simulink model "robot_rk"  (R2014b)
settings: Solver=ode45  StartTime=0.0  StopTime=10  FixedStep=1e-4  RelTol=1e-3
values from neighbouring files (symbols this model uses):
  robot_floor_friction_coeff = 0.6    [robot_init.m]
  robot_floor_position_gain = -1e5    (= -100000)    [robot_init.m]
  robot_floor_speed_gain = -1e3    (= -1000)    [robot_init.m]
  robot_gravity = [0 0 -9.80665]    [robot_init.m]
undefined symbols (not defined in the file or in its folder): CM730_acc_center, CM730_acc_gain, CM730_default, CM730_gyro_center, CM730_gyro_gain, CM730_sample_time, FSR_max, FSR_no_load, FSR_sample_time, FSR_scale, MX28_default, MX28_inertia, MX28_Te, X, Y, Z
libraries: sm_lib x158, fl_lib x128, nesl_utility x77
(part 6 of 6)

== system robot_rk/Right Leg/Floor model/Floor Model Front Right ==
  6-DOF Joint1 : sm_lib/Joints/6-DOF Joint  SenseConstraintForce=off  SenseConstraintForceX=off  SenseConstraintForceY=off  SenseConstraintForceZ=off  SenseConstraintTorque=off  SenseConstraintTorqueX=off  SenseConstraintTorqueY=off  SenseConstraintTorqueZ=off  SenseTotalForce=off  SenseTotalForceX=off  SenseTotalForceY=off  SenseTotalForceZ=off  SenseTotalTorque=off  SenseTotalTorqueX=off  SenseTotalTorqueY=off  SenseTotalTorqueZ=off  CompositeWrenchDir=FollowerOnBase  CompositeWrenchFrame=BaseFrame  PxEquilibriumPosition=0  PxEquilibriumPositionUnits=m  PxSpringStiffness=0  PxSpringStiffnessUnits=N/m  PxDampingCoefficient=0  PxDampingCoefficientUnits=N/(m/s)  PxTorqueActuationMode=InputTorque  PxMotionActuationMode=ComputedMotion  PxSensePosition=off  PxSenseVelocity=on  PxSenseAcceleration=off  PxSenseTorqueForce=off  PxPositionTargetValue=0  PxPositionTargetValueUnits=m  PxPositionTargetSpecify=off  PxPositionTargetPriority=High  PxVelocityTargetValue=0  PxVelocityTargetValueUnits=m/s  PxVelocityTargetSpecify=off  PxVelocityTargetPriority=High  PyEquilibriumPosition=0  PyEquilibriumPositionUnits=m  PySpringStiffness=0  PySpringStiffnessUnits=N/m  PyDampingCoefficient=0  PyDampingCoefficientUnits=N/(m/s)  PyTorqueActuationMode=InputTorque  PyMotionActuationMode=ComputedMotion  PySensePosition=off  PySenseVelocity=on  PySenseAcceleration=off  PySenseTorqueForce=off  PyPositionTargetValue=0  PyPositionTargetValueUnits=m  PyPositionTargetSpecify=off  PyPositionTargetPriority=High  PyVelocityTargetValue=0  PyVelocityTargetValueUnits=m/s  PyVelocityTargetSpecify=off  PyVelocityTargetPriority=High  PzEquilibriumPosition=0  PzEquilibriumPositionUnits=m  PzSpringStiffness=0  PzSpringStiffnessUnits=N/m  PzDampingCoefficient=0  PzDampingCoefficientUnits=N/(m/s)  PzTorqueActuationMode=InputTorque  PzMotionActuationMode=ComputedMotion  PzSensePosition=on  PzSenseVelocity=on  PzSenseAcceleration=off  PzSenseTorqueForce=off  PzPositionTargetValue=0  PzPositionTargetValueUnits=m  PzPositionTargetSpecify=off  PzPositionTargetPriority=High  PzVelocityTargetValue=0  PzVelocityTargetValueUnits=m/s  PzVelocityTargetSpecify=off  PzVelocityTargetPriority=High  SphDefPosRotationMethod=None  SphDefPosRotationAngleUnits=deg  SphDefPosRotationStandardAxis=+Z  SphDefPosRotationAngle=0.0  SphDefPosRotationArbitraryAxis=[0 0 1]  SphDefPosFollAlignAxisA=+X  SphDefPosBaseAlignAxisA=+Y  SphDefPosFollAlignAxisB=+Y  SphDefPosBaseAlignAxisB=+Z  SphDefPosRotationMatrix=[1 0 0; 0 1 0; 0 0 1]  SphEqPosRotationMethod=None  SphEqPosRotationAngleUnits=deg  SphEqPosRotationStandardAxis=+Z  SphEqPosRotationAngle=0.0  SphEqPosRotationArbitraryAxis=[0 0 1]  SphEqPosFollAlignAxisA=+X  SphEqPosBaseAlignAxisA=+Y  SphEqPosFollAlignAxisB=+Y  SphEqPosBaseAlignAxisB=+Z  SphEqPosRotationMatrix=[1 0 0; 0 1 0; 0 0 1]  SphSpringStiffness=0  SphSpringStiffnessUnits=N*m/deg  SphDampingCoefficient=0  SphDampingCoefficientUnits=N*m/(deg/s)  SphActuateTorqueX=off  SphActuateTorqueY=off  SphActuateTorqueZ=off  SphActuateTorque=off  SphTorqueActuationMode=NoTorque  SphMotionActuationMode=ComputedMotion  SphActuationFrame=BaseFrame  SphSensePosition=off  SphSenseVelocityX=off  SphSenseVelocityY=off  SphSenseVelocityZ=off  SphSenseVelocity=off  SphSenseAccelerationX=off  SphSenseAccelerationY=off  SphSenseAccelerationZ=off  SphSenseAcceleration=off  SphSenseTorqueX=off  SphSenseTorqueY=off  SphSenseTorqueZ=off  SphSenseTorqueForce=off  SphSensingFrame=BaseFrame  SphPositionTargetRotationMethod=None  SphPositionTargetRotationAngleUnits=deg  SphPositionTargetRotationStandardAxis=+Z  SphPositionTargetRotationAngle=0.0  SphPositionTargetRotationArbitraryAxis=[0 0 1]  SphPositionTargetFollAlignAxisA=+X  SphPositionTargetBaseAlignAxisA=+Y  SphPositionTargetFollAlignAxisB=+Y  SphPositionTargetBaseAlignAxisB=+Z  SphPositionTargetRotationMatrix=[1 0 0; 0 1 0; 0 0 1]  SphPositionTargetSpecify=off  SphPositionTargetPriority=High  SphVelocityTargetValue=[0 0 0]  SphVelocityTargetValueUnits=deg/s  SphVelocityTargetSpecify=off  SphVelocityTargetPriority=High  SphVelocityTargetInFollowerFrame=on  BlockFunction=simmechanics.library.joints.sixdof_joint
  Friction coeff : fl_lib/Physical Signals/Functions/PS Gain  gain=robot_floor_friction_coeff
  No friction : fl_lib/Physical Signals/Sources/PS Constant  constant=0
  PS Abs : fl_lib/Physical Signals/Nonlinear Operators/PS Abs
  PS-Simulink Converter : nesl_utility/PS-Simulink Converter  PhysicalDomain=network_engine_domain  SubClassName=ps_output  LeftPortType=input  RightPortType=output  PseudoPeriodic=off  Frequencies=[]  Unit=N  AffineConversion=off
  Saturation : Saturate  UpperLimit=+inf  LowerLimit=0
  Unary minus : fl_lib/Physical Signals/Functions/PS Gain  gain=-1
  X Lower Bound : fl_lib/Physical Signals/Nonlinear Operators/PS Max
  X Speed Gain : fl_lib/Physical Signals/Functions/PS Gain  gain=robot_floor_speed_gain
  X Switch : fl_lib/Physical Signals/Nonlinear Operators/PS Switch  Threshold=0
  X Upper Bound : fl_lib/Physical Signals/Nonlinear Operators/PS Min
  Y Lower Bound : fl_lib/Physical Signals/Nonlinear Operators/PS Max
  Y Speed Gain : fl_lib/Physical Signals/Functions/PS Gain  gain=robot_floor_speed_gain
  Y Switch : fl_lib/Physical Signals/Nonlinear Operators/PS Switch  Threshold=0
  Y Upper Bound : fl_lib/Physical Signals/Nonlinear Operators/PS Min
  Z Add : fl_lib/Physical Signals/Functions/PS Add
  Z Position Gain : fl_lib/Physical Signals/Functions/PS Gain  gain=robot_floor_position_gain
  Z Speed Gain : fl_lib/Physical Signals/Functions/PS Gain  gain=robot_floor_speed_gain
  Z Switch : fl_lib/Physical Signals/Nonlinear Operators/PS Switch  Threshold=0
  Contact : PMIOPort  Port=1  Side=Left
  Floor : PMIOPort  Port=2  Side=Right
  Z force : Outport
  wires:
  PS-Simulink Converter/1 -> Saturation/1
  Saturation/1 -> Z force/1
  connections:
  Floor/RConn1 -- 6-DOF Joint1/LConn1
  6-DOF Joint1/RConn1 -- Contact/RConn1
  No friction/RConn1 -- Y Switch/LConn1 -- Z Switch/LConn1 -- X Switch/LConn1
  Z Position Gain/RConn1 -- Z Add/LConn1
  Z Switch/LConn3 -- Z Add/RConn1 -- Friction coeff/LConn1 -- PS-Simulink Converter/LConn1
  Z Speed Gain/RConn1 -- Z Add/LConn2
  6-DOF Joint1/RConn5 -- Z Speed Gain/LConn1
  6-DOF Joint1/LConn4 -- Z Switch/RConn1
  Z Switch/LConn2 -- Z Position Gain/LConn1 -- 6-DOF Joint1/RConn4 -- X Switch/LConn2 -- Y Switch/LConn2
  Y Switch/RConn1 -- 6-DOF Joint1/LConn3
  Y Speed Gain/LConn1 -- 6-DOF Joint1/RConn3
  PS Abs/LConn1 -- Friction coeff/RConn1
  PS Abs/RConn1 -- Unary minus/LConn1 -- X Upper Bound/LConn2 -- Y Upper Bound/LConn2
  Y Upper Bound/RConn1 -- Y Lower Bound/LConn1
  Y Lower Bound/LConn2 -- Unary minus/RConn1 -- X Lower Bound/LConn2
  Y Lower Bound/RConn1 -- Y Switch/LConn3
  Y Upper Bound/LConn1 -- Y Speed Gain/RConn1
  X Speed Gain/LConn1 -- 6-DOF Joint1/RConn2
  X Upper Bound/LConn1 -- X Speed Gain/RConn1
  X Lower Bound/LConn1 -- X Upper Bound/RConn1
  X Switch/LConn3 -- X Lower Bound/RConn1
  X Switch/RConn1 -- 6-DOF Joint1/LConn2

== stateflow chart robot_rk/Right Kick ==
  settings: updateMethod=DISCRETE  sampleTime=MX28_Te
  state Initialization
    entry: Robot_Init();
    entry: delay = 0;
    during: delay = delay+1;
  state Right_Kick_0_State
    entry: Right_Kick_0();
    entry: delay = 0;
    during: delay = delay+1;
  state Right_Kick_6_State
    entry: Right_Kick_6()
    entry: delay = 0;
    during: delay = delay + 1;
  state Right_Kick_1_State
    entry: Right_Kick_1()
    entry: delay = 0;
    during: delay = delay + 1;
  state Right_Kick_5_State
    entry: Right_Kick_5()
    entry: delay = 0;
    during: delay = delay + 1;
  state Right_Kick_2_State
    entry: Right_Kick_2()
    entry: delay = 0;
    during: delay = delay + 1;
  state Right_Kick_4_State
    entry: Right_Kick_4()
    entry: delay = 0;
    during: delay = delay + 1;
  state Right_Kick_3_Delay
    entry: delay = 0;
    during: delay = delay + 1;
  state Right_Kick_3_State
    entry: Right_Kick_3()
    entry: delay = 0;
    during: delay = delay + 1;
  (default) -> Initialization
  Initialization -> Right_Kick_0_State : [delay >= 200]
  Right_Kick_6_State -> Right_Kick_0_State : [delay>=496]
  Right_Kick_0_State -> Right_Kick_1_State : [delay>=496]
  Right_Kick_5_State -> Right_Kick_6_State : [delay>=112]
  Right_Kick_1_State -> Right_Kick_2_State : [delay>=200]
  Right_Kick_4_State -> Right_Kick_5_State : [delay>=72]
  Right_Kick_2_State -> Right_Kick_3_Delay : [delay>=72]
  Right_Kick_3_Delay -> Right_Kick_3_State : [delay>=144]
  Right_Kick_3_State -> Right_Kick_4_State : [delay>=72]
  data: positions function_input int16 size=[1 20]; moving_time function_input double; MX28_ID1 data_store_memory; MX28_ID2 data_store_memory; MX28_ID3 data_store_memory; MX28_ID4 data_store_memory; MX28_ID5 data_store_memory; MX28_ID6 data_store_memory; MX28_ID7 data_store_memory; MX28_ID8 data_store_memory; MX28_ID9 data_store_memory; MX28_ID10 data_store_memory; MX28_ID11 data_store_memory; MX28_ID12 data_store_memory; MX28_ID13 data_store_memory; MX28_ID14 data_store_memory; MX28_ID15 data_store_memory; MX28_ID16 data_store_memory; MX28_ID17 data_store_memory; MX28_ID18 data_store_memory; MX28_ID19 data_store_memory; MX28_ID20 data_store_memory; MX28_default parameter Bus: MX28_bus; CM730_ID200 data_store_memory; CM730_default parameter Bus: CM730_bus; FSR_ID111 data_store_memory; FSR_ID112 data_store_memory; delay local int16 =0
  function Apply_Position_Speed(positions,moving_time):
    | function Apply_Position_Speed(positions,moving_time)
    | 
    | speed_ratio = 1024 / moving_time / 8;
    | 
    | MX28_ID1.moving_speed = abs(MX28_ID1.goal_position - positions(1)) * speed_ratio;
    | MX28_ID1.goal_position = positions(1);
    | 
    | MX28_ID2.moving_speed = abs(MX28_ID2.goal_position - positions(2)) * speed_ratio;
    | MX28_ID2.goal_position = positions(2);
    | 
    | MX28_ID3.moving_speed = abs(MX28_ID3.goal_position - positions(3)) * speed_ratio;
    | MX28_ID3.goal_position = positions(3);
    | 
    | MX28_ID4.moving_speed = abs(MX28_ID4.goal_position - positions(4)) * speed_ratio;
    | MX28_ID4.goal_position = positions(4);
    | 
    | MX28_ID5.moving_speed = abs(MX28_ID5.goal_position - positions(5)) * speed_ratio;
    | MX28_ID5.goal_position = positions(5);
    | 
    | MX28_ID6.moving_speed = abs(MX28_ID6.goal_position - positions(6)) * speed_ratio;
    | MX28_ID6.goal_position = positions(6);
    | 
    | MX28_ID7.moving_speed = abs(MX28_ID7.goal_position - positions(7)) * speed_ratio;
    | MX28_ID7.goal_position = positions(7);
    | 
    | MX28_ID8.moving_speed = abs(MX28_ID8.goal_position - positions(8)) * speed_ratio;
    | MX28_ID8.goal_position = positions(8);
    | 
    | MX28_ID9.moving_speed = abs(MX28_ID9.goal_position - positions(9)) * speed_ratio;
    | MX28_ID9.goal_position = positions(9);
    | 
    | MX28_ID10.moving_speed = abs(MX28_ID10.goal_position - positions(10)) * speed_ratio;
    | MX28_ID10.goal_position = positions(10);
    | 
    | MX28_ID11.moving_speed = abs(MX28_ID11.goal_position - positions(11)) * speed_ratio;
    | MX28_ID11.goal_position = positions(11);
    | 
    | MX28_ID12.moving_speed = abs(MX28_ID12.goal_position - positions(12)) * speed_ratio;
    | MX28_ID12.goal_position = positions(12);
    | 
    | MX28_ID13.moving_speed = abs(MX28_ID13.goal_position - positions(13)) * speed_ratio;
    | MX28_ID13.goal_position = positions(13);
    | 
    | MX28_ID14.moving_speed = abs(MX28_ID14.goal_position - positions(14)) * speed_ratio;
    | MX28_ID14.goal_position = positions(14);
    | 
    | MX28_ID15.moving_speed = abs(MX28_ID15.goal_position - positions(15)) * speed_ratio;
    | MX28_ID15.goal_position = positions(15);
    | 
    | MX28_ID16.moving_speed = abs(MX28_ID16.goal_position - positions(16)) * speed_ratio;
    | MX28_ID16.goal_position = positions(16);
    | 
    | MX28_ID17.moving_speed = abs(MX28_ID17.goal_position - positions(17)) * speed_ratio;
    | MX28_ID17.goal_position = positions(17);
    | 
    | MX28_ID18.moving_speed = abs(MX28_ID18.goal_position - positions(18)) * speed_ratio;
    | MX28_ID18.goal_position = positions(18);
    | 
    | MX28_ID19.moving_speed = abs(MX28_ID19.goal_position - positions(19)) * speed_ratio;
    | MX28_ID19.goal_position = positions(19);
    | 
    | MX28_ID20.moving_speed = abs(MX28_ID20.goal_position - positions(20)) * speed_ratio;
    | MX28_ID20.goal_position = positions(20);
  function Robot_Init:
    | function Robot_Init
    | 
    | global MX28_default
    | 
    | MX28_ID1.torque_enable = MX28_default.torque_enable;
    | MX28_ID1.D_gain        = MX28_default.D_gain;
    | MX28_ID1.I_gain        = MX28_default.I_gain;
    | MX28_ID1.P_gain        = MX28_default.P_gain;
    | MX28_ID1.goal_position = MX28_default.goal_position;
    | MX28_ID1.moving_speed  = MX28_default.moving_speed;
    | MX28_ID1.torque_limit  = MX28_default.torque_limit;
    | 
    | MX28_ID2.torque_enable = MX28_default.torque_enable;
    | MX28_ID2.D_gain        = MX28_default.D_gain;
    | MX28_ID2.I_gain        = MX28_default.I_gain;
    | MX28_ID2.P_gain        = MX28_default.P_gain;
    | MX28_ID2.goal_position = MX28_default.goal_position;
    | MX28_ID2.moving_speed  = MX28_default.moving_speed;
    | MX28_ID2.torque_limit  = MX28_default.torque_limit;
    | 
    | MX28_ID3.torque_enable = MX28_default.torque_enable;
    | MX28_ID3.D_gain        = MX28_default.D_gain;
    | MX28_ID3.I_gain        = MX28_default.I_gain;
    | MX28_ID3.P_gain        = MX28_default.P_gain;
    | MX28_ID3.goal_position = MX28_default.goal_position;
    | MX28_ID3.moving_speed  = MX28_default.moving_speed;
    | MX28_ID3.torque_limit  = MX28_default.torque_limit;
    | 
    | MX28_ID4.torque_enable = MX28_default.torque_enable;
    | MX28_ID4.D_gain        = MX28_default.D_gain;
    | MX28_ID4.I_gain        = MX28_default.I_gain;
    | MX28_ID4.P_gain        = MX28_default.P_gain;
    | MX28_ID4.goal_position = MX28_default.goal_position;
    | MX28_ID4.moving_speed  = MX28_default.moving_speed;
    | MX28_ID4.torque_limit  = MX28_default.torque_limit;
    | 
    | MX28_ID5.torque_enable = MX28_default.torque_enable;
    | MX28_ID5.D_gain        = MX28_default.D_gain;
    | MX28_ID5.I_gain        = MX28_default.I_gain;
    | MX28_ID5.P_gain        = MX28_default.P_gain;
    | MX28_ID5.goal_position = MX28_default.goal_position;
    | MX28_ID5.moving_speed  = MX28_default.moving_speed;
    | MX28_ID5.torque_limit  = MX28_default.torque_limit;
    | 
    | MX28_ID6.torque_enable = MX28_default.torque_enable;
    | MX28_ID6.D_gain        = MX28_default.D_gain;
    | MX28_ID6.I_gain        = MX28_default.I_gain;
    | MX28_ID6.P_gain        = MX28_default.P_gain;
    | MX28_ID6.goal_position = MX28_default.goal_position;
    | MX28_ID6.moving_speed  = MX28_default.moving_speed;
    | MX28_ID6.torque_limit  = MX28_default.torque_limit;
    | 
    | MX28_ID7.torque_enable = MX28_default.torque_enable;
    | MX28_ID7.D_gain        = MX28_default.D_gain;
    | MX28_ID7.I_gain        = MX28_default.I_gain;
    | MX28_ID7.P_gain        = MX28_default.P_gain;
    | MX28_ID7.goal_position = MX28_default.goal_position;
    | MX28_ID7.moving_speed  = MX28_default.moving_speed;
    | MX28_ID7.torque_limit  = MX28_default.torque_limit;
    | 
    | MX28_ID8.torque_enable = MX28_default.torque_enable;
    | MX28_ID8.D_gain        = MX28_default.D_gain;
    | MX28_ID8.I_gain        = MX28_default.I_gain;
    | MX28_ID8.P_gain        = MX28_default.P_gain;
    | MX28_ID8.goal_position = MX28_default.goal_position;
    | MX28_ID8.moving_speed  = MX28_default.moving_speed;
    | MX28_ID8.torque_limit  = MX28_default.torque_limit;
    | 
    | MX28_ID9.torque_enable = MX28_default.torque_enable;
    | MX28_ID9.D_gain        = MX28_default.D_gain;
    | MX28_ID9.I_gain        = MX28_default.I_gain;
    | MX28_ID9.P_gain        = MX28_default.P_gain;
    | MX28_ID9.goal_position = MX28_default.goal_position;
    | MX28_ID9.moving_speed  = MX28_default.moving_speed;
    | MX28_ID9.torque_limit  = MX28_default.torque_limit;
    | 
    | MX28_ID10.torque_enable = MX28_default.torque_enable;
    | MX28_ID10.D_gain        = MX28_default.D_gain;
    | MX28_ID10.I_gain        = MX28_default.I_gain;
    | MX28_ID10.P_gain        = MX28_default.P_gain;
    | MX28_ID10.goal_position = MX28_default.goal_position;
    | MX28_ID10.moving_speed  = MX28_default.moving_speed;
    | MX28_ID10.torque_limit  = MX28_default.torque_limit;
    | 
    | MX28_ID11.torque_enable = MX28_default.torque_enable;
    | MX28_ID11.D_gain        = MX28_default.D_gain;
    | MX28_ID11.I_gain        = MX28_default.I_gain;
    | MX28_ID11.P_gain        = MX28_default.P_gain;
    | MX28_ID11.goal_position = MX28_default.goal_position;
    | MX28_ID11.moving_speed  = MX28_default.moving_speed;
    | MX28_ID11.torque_limit  = MX28_default.torque_limit;
    | 
    | MX28_ID12.torque_enable = MX28_default.torque_enable;
    | MX28_ID12.D_gain        = MX28_default.D_gain;
    | MX28_ID12.I_gain        = MX28_default.I_gain;
    | MX28_ID12.P_gain        = MX28_default.P_gain;
    | MX28_ID12.goal_position = MX28_default.goal_position;
    | MX28_ID12.moving_speed  = MX28_default.moving_speed;
    | MX28_ID12.torque_limit  = MX28_default.torque_limit;
    | 
    | MX28_ID13.torque_enable = MX28_default.torque_enable;
    | MX28_ID13.D_gain        = MX28_default.D_gain;
    | MX28_ID13.I_gain        = MX28_default.I_gain;
    | MX28_ID13.P_gain        = MX28_default.P_gain;
    | MX28_ID13.goal_position = MX28_default.goal_position;
    | MX28_ID13.moving_speed  = MX28_default.moving_speed;
    | MX28_ID13.torque_limit  = MX28_default.torque_limit;
    | 
    | MX28_ID14.torque_enable = MX28_default.torque_enable;
    | MX28_ID14.D_gain        = MX28_default.D_gain;
    | MX28_ID14.I_gain        = MX28_default.I_gain;
    | MX28_ID14.P_gain        = MX28_default.P_gain;
    | MX28_ID14.goal_position = MX28_default.goal_position;
    | MX28_ID14.moving_speed  = MX28_default.moving_speed;
    | MX28_ID14.torque_limit  = MX28_default.torque_limit;
    | 
    | MX28_ID15.torque_enable = MX28_default.torque_enable;
    | MX28_ID15.D_gain        = MX28_default.D_gain;
    | MX28_ID15.I_gain        = MX28_default.I_gain;
    | MX28_ID15.P_gain        = uint8(64); %MX28_default.P_gain;
    | MX28_ID15.goal_position = MX28_default.goal_position;
    | MX28_ID15.moving_speed  = MX28_default.moving_speed;
    | MX28_ID15.torque_limit  = MX28_default.torque_limit;
    | 
    | MX28_ID16.torque_enable = MX28_default.torque_enable;
    | MX28_ID16.D_gain        = MX28_default.D_gain;
    | MX28_ID16.I_gain        = MX28_default.I_gain;
    | MX28_ID16.P_gain        = uint8(64); %MX28_default.P_gain;
    | MX28_ID16.goal_position = MX28_default.goal_position;
    | MX28_ID16.moving_speed  = MX28_default.moving_speed;
    | MX28_ID16.torque_limit  = MX28_default.torque_limit;
    | 
    | MX28_ID17.torque_enable = MX28_default.torque_enable;
    | MX28_ID17.D_gain        = MX28_default.D_gain;
    | MX28_ID17.I_gain        = MX28_default.I_gain;
    | MX28_ID17.P_gain        = MX28_default.P_gain;
    | MX28_ID17.goal_position = MX28_default.goal_position;
    | MX28_ID17.moving_speed  = MX28_default.moving_speed;
    | MX28_ID17.torque_limit  = MX28_default.torque_limit;
    | 
    | MX28_ID18.torque_enable = MX28_default.torque_enable;
    | MX28_ID18.D_gain        = MX28_default.D_gain;
    | MX28_ID18.I_gain        = MX28_default.I_gain;
    | MX28_ID18.P_gain        = MX28_default.P_gain;
    | MX28_ID18.goal_position = MX28_default.goal_position;
    | MX28_ID18.moving_speed  = MX28_default.moving_speed;
    | MX28_ID18.torque_limit  = MX28_default.torque_limit;
    | 
    | MX28_ID19.torque_enable = MX28_default.torque_enable;
    | MX28_ID19.D_gain        = MX28_default.D_gain;
    | MX28_ID19.I_gain        = MX28_default.I_gain;
    | MX28_ID19.P_gain        = MX28_default.P_gain;
    | MX28_ID19.goal_position = MX28_default.goal_position;
    | MX28_ID19.moving_speed  = MX28_default.moving_speed;
    | MX28_ID19.torque_limit  = MX28_default.torque_limit;
    | 
    | MX28_ID20.torque_enable = MX28_default.torque_enable;
    | MX28_ID20.D_gain        = MX28_default.D_gain;
    | MX28_ID20.I_gain        = MX28_default.I_gain;
    | MX28_ID20.P_gain        = MX28_default.P_gain;
    | MX28_ID20.goal_position = MX28_default.goal_position;
    | MX28_ID20.moving_speed  = MX28_default.moving_speed;
    | MX28_ID20.torque_limit  = MX28_default.torque_limit;
  function Right_Kick_0:
    | function Right_Kick_0
    | 
    | positions = [ 1498 ... 1
    |               2518 ... 2
    |               1845 ... 3
    |               2248 ... 4
    |               2381 ... 5
    |               1712 ... 6
    |               2048 ... 7
    |               2048 ... 8
    |               2052 ... 9
    |               2044 ... 10
    |               1637 ... 11
    |               2459 ... 12
    |               2653 ... 13
    |               1443 ... 14
    |               2389 ... 15
    |               1707 ... 16
    |               2057 ... 17
    |               2039 ... 18
    |               2048 ... 19
    |               2161 ];% 20
    | 
    | Apply_Position_Speed(int16(positions),496);
  function Right_Kick_1:
    | function Right_Kick_1
    | 
    | positions = [ 1407 ... 1
    |               2420 ... 2
    |               1837 ... 3
    |               2287 ... 4
    |               2383 ... 5
    |               1714 ... 6
    |               2050 ... 7
    |               2050 ... 8
    |               2057 ... 9
    |               2043 ... 10
    |               1637 ... 11
    |               2459 ... 12
    |               2646 ... 13
    |               1443 ... 14
    |               2389 ... 15
    |               1707 ... 16
    |               2203 ... 17
    |               2160 ... 18
    |               2050 ... 19
    |               2207 ];% 20
    | 
    | Apply_Position_Speed(int16(positions),200);
  function Right_Kick_2:
    | function Right_Kick_2
    | 
    | positions = [ 1407 ... 1
    |               2420 ... 2
    |               1837 ... 3
    |               2287 ... 4
    |               2383 ... 5
    |               1714 ... 6
    |               2050 ... 7
    |               2050 ... 8
    |               2123 ... 9
    |               2010 ... 10
    |               1434 ... 11
    |               2593 ... 12
    |               3020 ... 13
    |               1394 ... 14
    |               2533 ... 15
    |               1707 ... 16
    |               2203 ... 17
    |               2160 ... 18
    |               2050 ... 19
    |               2207 ];% 20
    | 
    | Apply_Position_Speed(int16(positions),72);
  function Right_Kick_3:
    | function Right_Kick_3
    | 
    | positions = [ 1340 ... 1
    |               2220 ... 2
    |               1804 ... 3
    |               2287 ... 4
    |               2050 ... 5
    |               1480 ... 6
    |               2050 ... 7
    |               2050 ... 8
    |               2123 ... 9
    |               2010 ... 10
    |               1164 ... 11
    |               2543 ... 12
    |               2387 ... 13
    |               1414 ... 14
    |               1794 ... 15
    |               1740 ... 16
    |               2157 ... 17
    |               2127 ... 18
    |               2050 ... 19
    |               2207 ];% 20
    | 
    | Apply_Position_Speed(int16(positions),72);
  function Right_Kick_4:
    | function Right_Kick_4
    | 
    | positions = [ 1407 ... 1
    |               2420 ... 2
    |               1837 ... 3
    |               2287 ... 4
    |               2383 ... 5
    |               1714 ... 6
    |               2050 ... 7
    |               2050 ... 8
    |               2123 ... 9
    |               2010 ... 10
    |               1284 ... 11
    |               2533 ... 12
    |               3020 ... 13
    |               1414 ... 14
    |               2533 ... 15
    |               1714 ... 16
    |               2203 ... 17
    |               2160 ... 18
    |               2050 ... 19
    |               2207 ];% 20
    | 
    | Apply_Position_Speed(int16(positions),72);
  function Right_Kick_5:
    | function Right_Kick_5
    | 
    | positions = [ 1498 ... 1
    |               2518 ... 2
    |               1845 ... 3
    |               2248 ... 4
    |               2381 ... 5
    |               1712 ... 6
    |               2048 ... 7
    |               2048 ... 8
    |               2052 ... 9
    |               2044 ... 10
    |               1637 ... 11
    |               2459 ... 12
    |               2653 ... 13
    |               1443 ... 14
    |               2389 ... 15
    |               1707 ... 16
    |               2057 ... 17
    |               2039 ... 18
    |               2048 ... 19
    |               2161 ];% 20
    | 
    | Apply_Position_Speed(int16(positions),112);
  function Right_Kick_6:
    | function Right_Kick_6
    | 
    | positions = [ 1498 ... 1
    |               2518 ... 2
    |               1845 ... 3
    |               2248 ... 4
    |               2381 ... 5
    |               1712 ... 6
    |               2048 ... 7
    |               2048 ... 8
    |               2052 ... 9
    |               2044 ... 10
    |               1637 ... 11
    |               2459 ... 12
    |               2653 ... 13
    |               1443 ... 14
    |               2389 ... 15
    |               1707 ... 16
    |               2057 ... 17
    |               2039 ... 18
    |               2048 ... 19
    |               2161 ];% 20
    | 
    | Apply_Position_Speed(int16(positions),496);

== stateflow chart robot_rk/Left Pass ==
  settings: updateMethod=DISCRETE  sampleTime=MX28_Te
  state Initialization
    entry: Left_Pass_6();
    entry: delay = 0;
    during: delay = delay+1;
  state Left_Pass_0_State
    entry: Left_Pass_0();
    entry: delay = 0;
    during: delay = delay+1;
  state Left_Pass_6_State
    entry: Left_Pass_6()
    entry: delay = 0;
    during: delay = delay + 1;
  state Left_Pass_1_State
    entry: Left_Pass_1()
    entry: delay = 0;
    during: delay = delay + 1;
  state Left_Pass_5_State
    entry: Left_Pass_5()
    entry: delay = 0;
    during: delay = delay + 1;
  state Left_Pass_2_State
    entry: Left_Pass_2()
    entry: delay = 0;
    during: delay = delay + 1;
  state Left_Pass_4_State
    entry: Left_Pass_4()
    entry: delay = 0;
    during: delay = delay + 1;
  state Left_Pass_3_Delay
    entry: delay = 0;
    during: delay = delay + 1;
  state Left_Pass_3_State
    entry: Left_Pass_3()
    entry: delay = 0;
    during: delay = delay + 1;
  (default) -> Initialization
  Initialization -> Left_Pass_0_State : [delay >= 200]
  Left_Pass_6_State -> Left_Pass_0_State : [delay>=72]
  Left_Pass_0_State -> Left_Pass_1_State : [delay>=200]
  Left_Pass_5_State -> Left_Pass_6_State : [delay>=200]
  Left_Pass_1_State -> Left_Pass_2_State : [delay>=72]
  Left_Pass_4_State -> Left_Pass_5_State : [delay>=72]
  Left_Pass_2_State -> Left_Pass_3_Delay : [delay>=72]
  Left_Pass_3_Delay -> Left_Pass_3_State : [delay>=96]
  Left_Pass_3_State -> Left_Pass_4_State : [delay>=72]
  data: positions function_input int16 size=[1 20]; moving_time function_input double; MX28_ID1 data_store_memory; MX28_ID2 data_store_memory; MX28_ID3 data_store_memory; MX28_ID4 data_store_memory; MX28_ID5 data_store_memory; MX28_ID6 data_store_memory; MX28_ID7 data_store_memory; MX28_ID8 data_store_memory; MX28_ID9 data_store_memory; MX28_ID10 data_store_memory; MX28_ID11 data_store_memory; MX28_ID12 data_store_memory; MX28_ID13 data_store_memory; MX28_ID14 data_store_memory; MX28_ID15 data_store_memory; MX28_ID16 data_store_memory; MX28_ID17 data_store_memory; MX28_ID18 data_store_memory; MX28_ID19 data_store_memory; MX28_ID20 data_store_memory; MX28_default parameter Bus: MX28_bus; CM730_ID200 data_store_memory; CM730_default parameter Bus: CM730_bus; FSR_ID111 data_store_memory; FSR_ID112 data_store_memory; delay local int16 =0
  function Apply_Position_Speed(positions,moving_time):
    | function Apply_Position_Speed(positions,moving_time)
    | 
    | speed_ratio = 1024 / moving_time / 8;
    | 
    | MX28_ID1.moving_speed = min_max(abs(MX28_ID1.goal_position - positions(1)) * speed_ratio);
    | MX28_ID1.goal_position = positions(1);
    | 
    | MX28_ID2.moving_speed = min_max(abs(MX28_ID2.goal_position - positions(2)) * speed_ratio);
    | MX28_ID2.goal_position = positions(2);
    | 
    | MX28_ID3.moving_speed = min_max(abs(MX28_ID3.goal_position - positions(3)) * speed_ratio);
    | MX28_ID3.goal_position = positions(3);
    | 
    | MX28_ID4.moving_speed = min_max(abs(MX28_ID4.goal_position - positions(4)) * speed_ratio);
    | MX28_ID4.goal_position = positions(4);
    | 
    | MX28_ID5.moving_speed = min_max(abs(MX28_ID5.goal_position - positions(5)) * speed_ratio);
    | MX28_ID5.goal_position = positions(5);
    | 
    | MX28_ID6.moving_speed = min_max(abs(MX28_ID6.goal_position - positions(6)) * speed_ratio);
    | MX28_ID6.goal_position = positions(6);
    | 
    | MX28_ID7.moving_speed = min_max(abs(MX28_ID7.goal_position - positions(7)) * speed_ratio);
    | MX28_ID7.goal_position = positions(7);
    | 
    | MX28_ID8.moving_speed = min_max(abs(MX28_ID8.goal_position - positions(8)) * speed_ratio);
    | MX28_ID8.goal_position = positions(8);
    | 
    | MX28_ID9.moving_speed = min_max(abs(MX28_ID9.goal_position - positions(9)) * speed_ratio);
    | MX28_ID9.goal_position = positions(9);
    | 
    | MX28_ID10.moving_speed = min_max(abs(MX28_ID10.goal_position - positions(10)) * speed_ratio);
    | MX28_ID10.goal_position = positions(10);
    | 
    | MX28_ID11.moving_speed = min_max(abs(MX28_ID11.goal_position - positions(11)) * speed_ratio);
    | MX28_ID11.goal_position = positions(11);
    | 
    | MX28_ID12.moving_speed = min_max(abs(MX28_ID12.goal_position - positions(12)) * speed_ratio);
    | MX28_ID12.goal_position = positions(12);
    | 
    | MX28_ID13.moving_speed = min_max(abs(MX28_ID13.goal_position - positions(13)) * speed_ratio);
    | MX28_ID13.goal_position = positions(13);
    | 
    | MX28_ID14.moving_speed = min_max(abs(MX28_ID14.goal_position - positions(14)) * speed_ratio);
    | MX28_ID14.goal_position = positions(14);
    | 
    | MX28_ID15.moving_speed = min_max(abs(MX28_ID15.goal_position - positions(15)) * speed_ratio);
    | MX28_ID15.goal_position = positions(15);
    | 
    | MX28_ID16.moving_speed = min_max(abs(MX28_ID16.goal_position - positions(16)) * speed_ratio);
    | MX28_ID16.goal_position = positions(16);
    | 
    | MX28_ID17.moving_speed = min_max(abs(MX28_ID17.goal_position - positions(17)) * speed_ratio);
    | MX28_ID17.goal_position = positions(17);
    | 
    | MX28_ID18.moving_speed = min_max(abs(MX28_ID18.goal_position - positions(18)) * speed_ratio);
    | MX28_ID18.goal_position = positions(18);
    | 
    | MX28_ID19.moving_speed = min_max(abs(MX28_ID19.goal_position - positions(19)) * speed_ratio);
    | MX28_ID19.goal_position = positions(19);
    | 
    | MX28_ID20.moving_speed = min_max(abs(MX28_ID20.goal_position - positions(20)) * speed_ratio);
    | MX28_ID20.goal_position = positions(20);
    | 
    | function v = min_max(p)
    | 
    | v = min(max(p,0),1023);
  function Robot_Init:
    | function Robot_Init
    | 
    | global MX28_default
    | 
    | MX28_ID1.torque_enable = MX28_default.torque_enable;
    | MX28_ID1.D_gain        = MX28_default.D_gain;
    | MX28_ID1.I_gain        = MX28_default.I_gain;
    | MX28_ID1.P_gain        = MX28_default.P_gain;
    | MX28_ID1.goal_position = MX28_default.goal_position;
    | MX28_ID1.moving_speed  = MX28_default.moving_speed;
    | MX28_ID1.torque_limit  = MX28_default.torque_limit;
    | 
    | MX28_ID2.torque_enable = MX28_default.torque_enable;
    | MX28_ID2.D_gain        = MX28_default.D_gain;
    | MX28_ID2.I_gain        = MX28_default.I_gain;
    | MX28_ID2.P_gain        = MX28_default.P_gain;
    | MX28_ID2.goal_position = MX28_default.goal_position;
    | MX28_ID2.moving_speed  = MX28_default.moving_speed;
    | MX28_ID2.torque_limit  = MX28_default.torque_limit;
    | 
    | MX28_ID3.torque_enable = MX28_default.torque_enable;
    | MX28_ID3.D_gain        = MX28_default.D_gain;
    | MX28_ID3.I_gain        = MX28_default.I_gain;
    | MX28_ID3.P_gain        = MX28_default.P_gain;
    | MX28_ID3.goal_position = MX28_default.goal_position;
    | MX28_ID3.moving_speed  = MX28_default.moving_speed;
    | MX28_ID3.torque_limit  = MX28_default.torque_limit;
    | 
    | MX28_ID4.torque_enable = MX28_default.torque_enable;
    | MX28_ID4.D_gain        = MX28_default.D_gain;
    | MX28_ID4.I_gain        = MX28_default.I_gain;
    | MX28_ID4.P_gain        = MX28_default.P_gain;
    | MX28_ID4.goal_position = MX28_default.goal_position;
    | MX28_ID4.moving_speed  = MX28_default.moving_speed;
    | MX28_ID4.torque_limit  = MX28_default.torque_limit;
    | 
    | MX28_ID5.torque_enable = MX28_default.torque_enable;
    | MX28_ID5.D_gain        = MX28_default.D_gain;
    | MX28_ID5.I_gain        = MX28_default.I_gain;
    | MX28_ID5.P_gain        = MX28_default.P_gain;
    | MX28_ID5.goal_position = MX28_default.goal_position;
    | MX28_ID5.moving_speed  = MX28_default.moving_speed;
    | MX28_ID5.torque_limit  = MX28_default.torque_limit;
    | 
    | MX28_ID6.torque_enable = MX28_default.torque_enable;
    | MX28_ID6.D_gain        = MX28_default.D_gain;
    | MX28_ID6.I_gain        = MX28_default.I_gain;
    | MX28_ID6.P_gain        = MX28_default.P_gain;
    | MX28_ID6.goal_position = MX28_default.goal_position;
    | MX28_ID6.moving_speed  = MX28_default.moving_speed;
    | MX28_ID6.torque_limit  = MX28_default.torque_limit;
    | 
    | MX28_ID7.torque_enable = MX28_default.torque_enable;
    | MX28_ID7.D_gain        = MX28_default.D_gain;
    | MX28_ID7.I_gain        = MX28_default.I_gain;
    | MX28_ID7.P_gain        = MX28_default.P_gain;
    | MX28_ID7.goal_position = MX28_default.goal_position;
    | MX28_ID7.moving_speed  = MX28_default.moving_speed;
    | MX28_ID7.torque_limit  = MX28_default.torque_limit;
    | 
    | MX28_ID8.torque_enable = MX28_default.torque_enable;
    | MX28_ID8.D_gain        = MX28_default.D_gain;
    | MX28_ID8.I_gain        = MX28_default.I_gain;
    | MX28_ID8.P_gain        = MX28_default.P_gain;
    | MX28_ID8.goal_position = MX28_default.goal_position;
    | MX28_ID8.moving_speed  = MX28_default.moving_speed;
    | MX28_ID8.torque_limit  = MX28_default.torque_limit;
    | 
    | MX28_ID9.torque_enable = MX28_default.torque_enable;
    | MX28_ID9.D_gain        = MX28_default.D_gain;
    | MX28_ID9.I_gain        = MX28_default.I_gain;
    | MX28_ID9.P_gain        = MX28_default.P_gain;
    | MX28_ID9.goal_position = MX28_default.goal_position;
    | MX28_ID9.moving_speed  = MX28_default.moving_speed;
    | MX28_ID9.torque_limit  = MX28_default.torque_limit;
    | 
    | MX28_ID10.torque_enable = MX28_default.torque_enable;
    | MX28_ID10.D_gain        = MX28_default.D_gain;
    | MX28_ID10.I_gain        = MX28_default.I_gain;
    | MX28_ID10.P_gain        = MX28_default.P_gain;
    | MX28_ID10.goal_position = MX28_default.goal_position;
    | MX28_ID10.moving_speed  = MX28_default.moving_speed;
    | MX28_ID10.torque_limit  = MX28_default.torque_limit;
    | 
    | MX28_ID11.torque_enable = MX28_default.torque_enable;
    | MX28_ID11.D_gain        = MX28_default.D_gain;
    | MX28_ID11.I_gain        = MX28_default.I_gain;
    | MX28_ID11.P_gain        = MX28_default.P_gain;
    | MX28_ID11.goal_position = MX28_default.goal_position;
    | MX28_ID11.moving_speed  = MX28_default.moving_speed;
    | MX28_ID11.torque_limit  = MX28_default.torque_limit;
    | 
    | MX28_ID12.torque_enable = MX28_default.torque_enable;
    | MX28_ID12.D_gain        = MX28_default.D_gain;
    | MX28_ID12.I_gain        = MX28_default.I_gain;
    | MX28_ID12.P_gain        = MX28_default.P_gain;
    | MX28_ID12.goal_position = MX28_default.goal_position;
    | MX28_ID12.moving_speed  = MX28_default.moving_speed;
    | MX28_ID12.torque_limit  = MX28_default.torque_limit;
    | 
    | MX28_ID13.torque_enable = MX28_default.torque_enable;
    | MX28_ID13.D_gain        = MX28_default.D_gain;
    | MX28_ID13.I_gain        = MX28_default.I_gain;
    | MX28_ID13.P_gain        = MX28_default.P_gain;
    | MX28_ID13.goal_position = MX28_default.goal_position;
    | MX28_ID13.moving_speed  = MX28_default.moving_speed;
    | MX28_ID13.torque_limit  = MX28_default.torque_limit;
    | 
    | MX28_ID14.torque_enable = MX28_default.torque_enable;
    | MX28_ID14.D_gain        = MX28_default.D_gain;
    | MX28_ID14.I_gain        = MX28_default.I_gain;
    | MX28_ID14.P_gain        = MX28_default.P_gain;
    | MX28_ID14.goal_position = MX28_default.goal_position;
    | MX28_ID14.moving_speed  = MX28_default.moving_speed;
    | MX28_ID14.torque_limit  = MX28_default.torque_limit;
    | 
    | MX28_ID15.torque_enable = MX28_default.torque_enable;
    | MX28_ID15.D_gain        = MX28_default.D_gain;
    | MX28_ID15.I_gain        = MX28_default.I_gain;
    | MX28_ID15.P_gain        = uint8(64); %MX28_default.P_gain;
    | MX28_ID15.goal_position = MX28_default.goal_position;
    | MX28_ID15.moving_speed  = MX28_default.moving_speed;
    | MX28_ID15.torque_limit  = MX28_default.torque_limit;
    | 
    | MX28_ID16.torque_enable = MX28_default.torque_enable;
    | MX28_ID16.D_gain        = MX28_default.D_gain;
    | MX28_ID16.I_gain        = MX28_default.I_gain;
    | MX28_ID16.P_gain        = uint8(64); %MX28_default.P_gain;
    | MX28_ID16.goal_position = MX28_default.goal_position;
    | MX28_ID16.moving_speed  = MX28_default.moving_speed;
    | MX28_ID16.torque_limit  = MX28_default.torque_limit;
    | 
    | MX28_ID17.torque_enable = MX28_default.torque_enable;
    | MX28_ID17.D_gain        = MX28_default.D_gain;
    | MX28_ID17.I_gain        = MX28_default.I_gain;
    | MX28_ID17.P_gain        = MX28_default.P_gain;
    | MX28_ID17.goal_position = MX28_default.goal_position;
    | MX28_ID17.moving_speed  = MX28_default.moving_speed;
    | MX28_ID17.torque_limit  = MX28_default.torque_limit;
    | 
    | MX28_ID18.torque_enable = MX28_default.torque_enable;
    | MX28_ID18.D_gain        = MX28_default.D_gain;
    | MX28_ID18.I_gain        = MX28_default.I_gain;
    | MX28_ID18.P_gain        = MX28_default.P_gain;
    | MX28_ID18.goal_position = MX28_default.goal_position;
    | MX28_ID18.moving_speed  = MX28_default.moving_speed;
    | MX28_ID18.torque_limit  = MX28_default.torque_limit;
    | 
    | MX28_ID19.torque_enable = MX28_default.torque_enable;
    | MX28_ID19.D_gain        = MX28_default.D_gain;
    | MX28_ID19.I_gain        = MX28_default.I_gain;
    | MX28_ID19.P_gain        = MX28_default.P_gain;
    | MX28_ID19.goal_position = MX28_default.goal_position;
    | MX28_ID19.moving_speed  = MX28_default.moving_speed;
    | MX28_ID19.torque_limit  = MX28_default.torque_limit;
    | 
    | MX28_ID20.torque_enable = MX28_default.torque_enable;
    | MX28_ID20.D_gain        = MX28_default.D_gain;
    | MX28_ID20.I_gain        = MX28_default.I_gain;
    | MX28_ID20.P_gain        = MX28_default.P_gain;
    | MX28_ID20.goal_position = MX28_default.goal_position;
    | MX28_ID20.moving_speed  = MX28_default.moving_speed;
    | MX28_ID20.torque_limit  = MX28_default.torque_limit;
  function Left_Pass_0:
    | function Left_Pass_0
    | 
    | positions = [ 1670 ...
    | 2850 ...
    | 1804 ...
    | 2253 ...
    | 2377 ...
    | 2040 ...
    | 2040 ...
    | 2040 ...
    | 2047 ...
    | 2033 ...
    | 1524 ...
    | 2557 ...
    | 2677 ...
    | 1404 ...
    | 2357 ...
    | 1724 ...
    | 1947 ...
    | 1800 ...
    | 2050 ...
    | 2507 ...
    |  ];% 20
    | 
    | Apply_Position_Speed(int16(positions),200);
  function Left_Pass_1:
    | function Left_Pass_1
    | 
    | positions = [ 1670 ...
    | 2950 ...
    | 1804 ...
    | 2187 ...
    | 2377 ...
    | 2040 ...
    | 2040 ...
    | 1707 ...
    | 2080 ...
    | 1967 ...
    | 1457 ...
    | 2657 ...
    | 2677 ...
    | 1071 ...
    | 2357 ...
    | 1557 ...
    | 1947 ...
    | 1867 ...
    | 2050 ...
    | 2507 ...
    |  ];% 20
    | 
    | Apply_Position_Speed(int16(positions),72);
  function Left_Pass_2:
    | function Left_Pass_2
    | 
    | positions = [ 1870 ...
    | 2916 ...
    | 1804 ...
    | 2287 ...
    | 2610 ...
    | 2040 ...
    | 2040 ...
    | 1640 ...
    | 2080 ...
    | 2067 ...
    | 1557 ...
    | 2757 ...
    | 2677 ...
    | 1704 ...
    | 2340 ...
    | 2257 ...
    | 1947 ...
    | 1934 ...
    | 2050 ...
    | 2507 ...
    |  ];% 20
    | 
    | Apply_Position_Speed(int16(positions),72);
  function Left_Pass_3:
    | function Left_Pass_3
    | 
    | positions = [ 1870 ...
    | 3083 ...
    | 1804 ...
    | 2287 ...
    | 2610 ...
    | 2040 ...
    | 2040 ...
    | 1740 ...
    | 2080 ...
    | 2467 ...
    | 1557 ...
    | 2757 ...
    | 2677 ...
    | 1704 ...
    | 2340 ...
    | 2257 ...
    | 1947 ...
    | 1934 ...
    | 2050 ...
    | 2507 ...
    |  ];% 20
    | 
    | Apply_Position_Speed(int16(positions),72);
  function Left_Pass_4:
    | function Left_Pass_4
    | 
    | positions = [ 1870 ...
    | 2916 ...
    | 1804 ...
    | 2287 ...
    | 2610 ...
    | 2040 ...
    | 2040 ...
    | 1640 ...
    | 2080 ...
    | 2067 ...
    | 1557 ...
    | 2757 ...
    | 2677 ...
    | 1704 ...
    | 2340 ...
    | 2257 ...
    | 1947 ...
    | 1934 ...
    | 2050 ...
    | 2507 ...
    |  ];% 20
    | 
    | Apply_Position_Speed(int16(positions),72);
  function Left_Pass_5:
    | function Left_Pass_5
    | 
    | positions = [ 1570 ...
    | 2583 ...
    | 1804 ...
    | 2253 ...
    | 2377 ...
    | 1707 ...
    | 2040 ...
    | 2040 ...
    | 2080 ...
    | 2000 ...
    | 1524 ...
    | 2723 ...
    | 2677 ...
    | 1071 ...
    | 2357 ...
    | 1557 ...
    | 1964 ...
    | 1934 ...
    | 2050 ...
    | 2507 ...
    |  ];% 20
    | 
    | Apply_Position_Speed(int16(positions),200);
  function Left_Pass_6:
    | function Left_Pass_6
    | 
    | positions = [ 1500 ...
    | 2520 ...
    | 1837 ...
    | 2287 ...
    | 2383 ...
    | 1714 ...
    | 2050 ...
    | 2050 ...
    | 2057 ...
    | 2043 ...
    | 1534 ...
    | 2567 ...
    | 2687 ...
    | 1414 ...
    | 2367 ...
    | 1734 ...
    | 2057 ...
    | 2043 ...
    | 2050 ...
    | 2507 ...
    |  ];% 20
    | 
    | Apply_Position_Speed(int16(positions),72);
